simulink model "ScalerCalc"  (R2021a)
settings: Solver=FixedStepDiscrete  StartTime=0.0  StopTime=10.0  RelTol=1e-3  EnableMultiTasking=on
libraries: simulink x2
settings Model: Creator=Mina  LastModifiedBy=Mina
settings DataIOCC: ReturnWorkspaceOutputs=off
settings OptimizationCC: DefaultParameterBehavior=Inlined  InlineInvariantSignals=on  EnableMemcpy=off  LifeSpan=1  EfficientTunableParamExpr=on
settings DebuggingCC: UnderspecifiedInitializationDetection=Classic  MergeDetectMultiDrivingBlocksExec=none  SFMachineParentedDataDiag=warning  ArithmeticOperatorsInVariantConditions=warning
settings ModelReferenceCC: PropagateSignalLabelsOutOfModel=off
settings SFSimCC: MATLABDynamicMemAlloc=off  CustomCodeUndefinedFunction=UseInterfaceOnly
settings RTWCC: SystemTargetFile=ert.tlc  GenCodeOnly=on  TemplateMakefile=ert_default_tmf  GenerateReport=on  IncludeHyperlinkInReport=on  LaunchReport=on  GenerateTraceInfo=on  GenerateTraceReport=on  GenerateTraceReportSl=on  GenerateTraceReportSf=on  GenerateTraceReportEml=on
settings CodeAppCC: ForceParamTrailComments=on  IgnoreCustomStorageClasses=off  OperatorAnnotations=on  SimulinkDataObjDesc=on  SFDataObjDesc=on  MATLABFcnDesc=on  InsertBlockDesc=on  StateflowObjectComments=on  MATLABSourceComments=on
settings ERTTargetCC: MultiwordLength=2048  GenerateSampleERTMain=on  InlinedParameterPlacement=NonHierarchical  ERTCustomFileTemplate=example_file_process.tlc

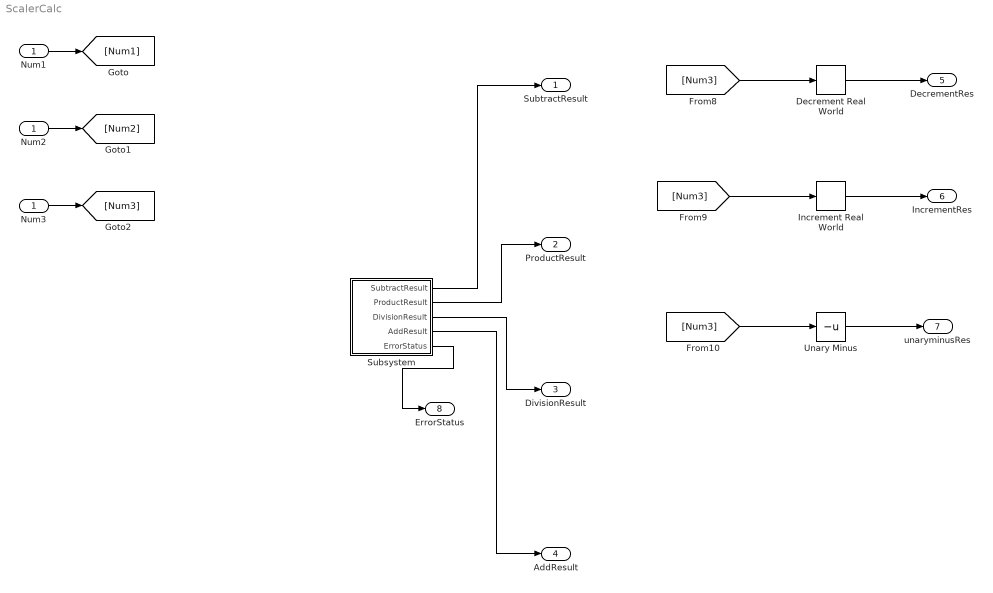
== system ScalerCalc ==
  Num1 : Inport  OutDataTypeStr=int8
  Decrement Real World : simulink/Additional Math & Discrete/Additional Math: Increment - Decrement/Decrement Real World
      settings: SourceProductBaseCode=SL
  Increment Real World : simulink/Additional Math & Discrete/Additional Math: Increment - Decrement/Increment Real World
      settings: SourceProductBaseCode=SL
  Num2 : InportShadow  OutDataTypeStr=int8
  Num3 : InportShadow  OutDataTypeStr=int8
  Subsystem : Subsystem  TreatAsAtomicUnit=on
      settings: RTWFcnNameOpts=Use subsystem name  RTWFileNameOpts=Use subsystem name
  Unary Minus : UnaryMinus
  SubtractResult : Outport
  ProductResult : Outport  Port=2
  DivisionResult : Outport  Port=3
  AddResult : Outport  Port=4
  DecrementRes : Outport  Port=5
  IncrementRes : Outport  Port=6
  unaryminusRes : Outport  Port=7
  ErrorStatus : Outport  Port=8
  wires:
  Num1/1 -> [Num1]
  Num2/1 -> [Num2]
  Num3/1 -> [Num3]
  Unary Minus/1 -> unaryminusRes/1
  [Num3] -> Unary Minus/1
  [Num3] -> Increment Real World/1
  [Num3] -> Decrement Real World/1
  Decrement Real World/1 -> DecrementRes/1
  Increment Real World/1 -> IncrementRes/1
  Subsystem/1(SubtractResult) -> SubtractResult/1
  Subsystem/2(ProductResult) -> ProductResult/1
  Subsystem/3(DivisionResult) -> DivisionResult/1
  Subsystem/4(AddResult) -> AddResult/1
  Subsystem/5(ErrorStatus) -> ErrorStatus/1

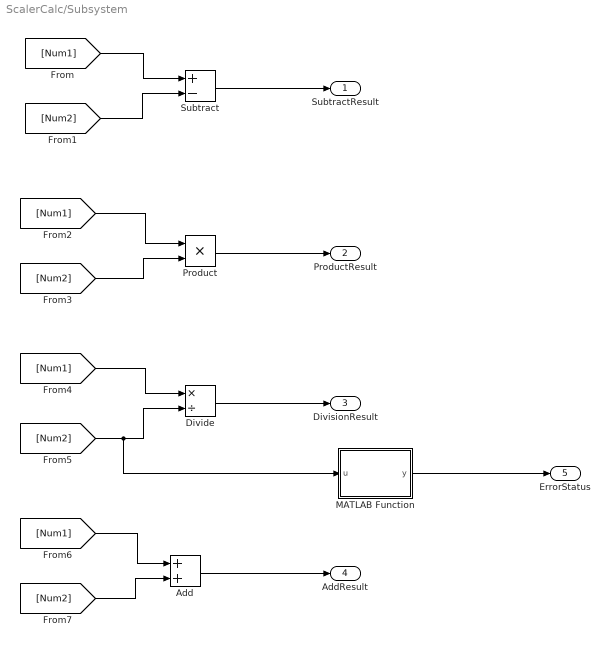
== system ScalerCalc/Subsystem ==
  Add : Sum  OutDataTypeStr=uint16
  Divide : Product  Inputs=*/  OutDataTypeStr=uint16
  MATLAB Function : MATLAB Function  TreatAsAtomicUnit=on
  Product : Product  OutDataTypeStr=uint16
  Subtract : Sum  Inputs=+-  OutDataTypeStr=uint16
  SubtractResult : Outport
  ProductResult : Outport  Port=2
  DivisionResult : Outport  Port=3
  AddResult : Outport  Port=4
  ErrorStatus : Outport  Port=5
  wires:
  [Num1] -> Subtract/1
  Divide/1 -> DivisionResult/1
  [Num1] -> Divide/1
  Subtract/1 -> SubtractResult/1
  [Num2] -> Product/2
  Product/1 -> ProductResult/1
  [Num1] -> Product/1
  [Num2] -> Add/2
  [Num2] -> Subtract/2
  [Num2] -> MATLAB Function/1(u), Divide/2
  Add/1 -> AddResult/1
  [Num1] -> Add/1
  MATLAB Function/1(y) -> ErrorStatus/1

== matlab function ScalerCalc/Subsystem/MATLAB Function ==
  data: u input; y output
function y = fcn(u)

if u==0
    y=1;
else
    y=0;
end
